simulink model "LQG_test"  (R2015a)
settings: Solver=ode5  StartTime=0.0  StopTime=14  FixedStep=1e-4  RelTol=1e-3
values from neighbouring files (symbols this model uses):
  Ak = [815.666686466 -247.565739392 216455.990143 -40009.9793013 101833.013371 56966.4369443 -260.344441883 79.637972257 -70891.4834769 12846.1132956 -26185.98219 -17361.2721412 ... (36 elements, 6x6)]    [controller.mat]    (also in main_matlab_step1.m = rlqg.A)
  Ap = Ap(1:nn,1:nn)    [main_matlab_step1.m]    (also in plant.mat = [-0.773996386153 -96.4009703983 0 0 0 0 96.979553948 -1.6354)
  Bk = [-8.44020481469 2.14766413524 104.526982436 -93.1116400352 -68.3572551974 -11.8211224455]    [controller.mat]    (also in main_matlab_step1.m = rlqg.B)
  Bp = [-0.230745598618  -0.153904745996; 0.0612777559553  0.0606173681668; -25.0923163191  13.5416143638; 4.01556833701  -3.21559278869; -4.90371370695  20.5766878764; -5.44248661254  6.08611624326]    [plant.mat]
  Ck = [-6676.24518167  2388.66763685  162.329744068  -97.9536908458  -117.882548171  -121.1765543; 3434.83172263  -735.119667317  -67.5589205763  -7.32978906487  3.89518348807  52.6776382701]    [controller.mat]    (also in main_matlab_step1.m = rlqg.C)
  Cp = [-23.1554338545 9.56281796835 0.435674513054 -0.46619419818 -0.57533927079 -0.316369760482]    [plant.mat]
  Dk = [0 0]    [controller.mat]    (also in main_matlab_step1.m = rlqg.D)
  Hp = [0.258916103899 0.10195659276 -1.80129126805 -4.56185147008 25.0926976513 -19.7319673467]    [plant.mat]
libraries: simulink x1
settings Model: Creator=p4wp4w  LastModifiedBy=p4wp4w

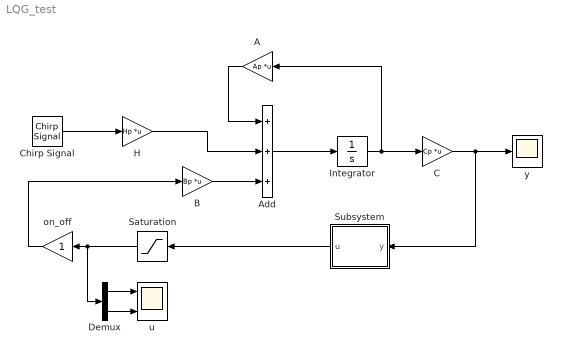
== system LQG_test ==
  A : Gain  Gain=Ap  Multiplication=Matrix(K*u)
  Add : Sum  Inputs=+++
  B : Gain  Gain=Bp  Multiplication=Matrix(K*u)
  C : Gain  Gain=Cp  Multiplication=Matrix(K*u)
  Chirp Signal : simulink/Sources/Chirp Signal  f1=0.1  T=14  f2=140
  Demux : Demux  Outputs=2
  H : Gain  Gain=Hp  Multiplication=Matrix(K*u)
  Integrator : Integrator
  Saturation : Saturate  UpperLimit=1.5  LowerLimit=-1.5
  Subsystem : Subsystem
  on_off : Gain
  u : Scope  NumInputPorts=2
      settings: YMin=-5~-5  YMax=5~5
  y : Scope
      settings: YMin=-0.03  YMax=0.03
  wires:
  Add/1 -> Integrator/1
  A/1 -> Add/1
  B/1 -> Add/3
  Integrator/1 -> C/1, A/1
  H/1 -> Add/2
  Chirp Signal/1 -> H/1
  on_off/1 -> B/1
  Demux/1 -> u/1
  Demux/2 -> u/2
  Saturation/1 -> Demux/1, on_off/1
  C/1 -> Subsystem/1(y), y/1
  Subsystem/1("u ") -> Saturation/1

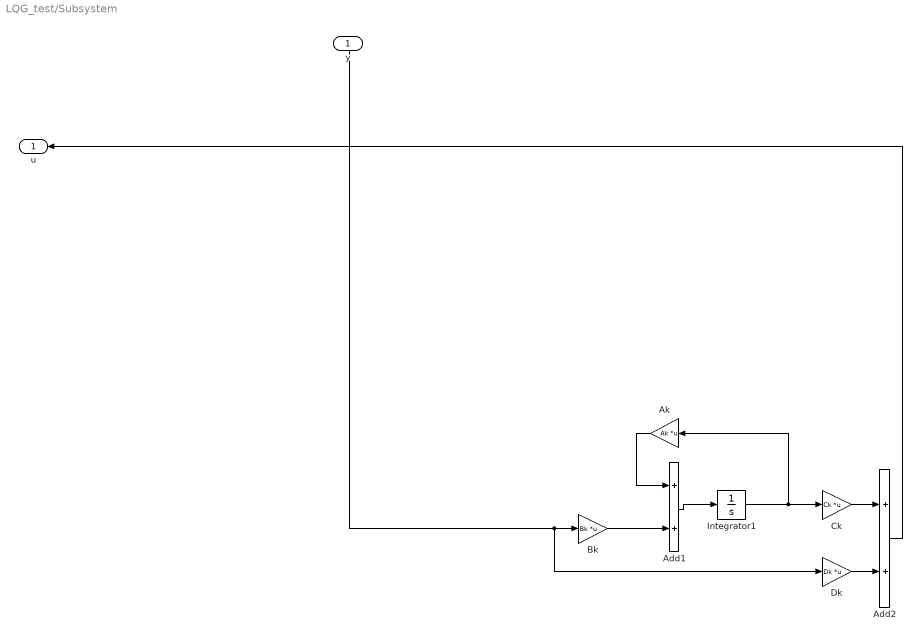
== system LQG_test/Subsystem ==
  y : Inport
  Add1 : Sum
  Add2 : Sum
  Ak : Gain  Gain=Ak  Multiplication=Matrix(K*u)
  Bk : Gain  Gain=Bk  Multiplication=Matrix(K*u)
  Ck : Gain  Gain=Ck  Multiplication=Matrix(K*u)
  Dk : Gain  Gain=Dk  Multiplication=Matrix(K*u)
  Integrator1 : Integrator
  "u " : Outport
  wires:
  y/1 -> Bk/1, Dk/1
  Add2/1 -> "u "/1
  Bk/1 -> Add1/2
  Ak/1 -> Add1/1
  Add1/1 -> Integrator1/1
  Dk/1 -> Add2/2
  Integrator1/1 -> Ck/1, Ak/1
  Ck/1 -> Add2/1
